simulink model "orion_casestudy_16"  (R2023a)
settings: Solver=VariableStepAuto  StartTime=0.0  StopTime=30  RelTol=1e-3
InitFcn:
  | RandStream.setGlobalStream(RandStream('mt19937ar','seed',sum(100*clock)));
undefined symbols (not defined in the file or in its folder): m, n
(part 2 of 4)

== stateflow chart orion_casestudy_16/Slave3 ==
  settings: updateMethod=CONTINUOUS
  state Connected
    entry:
    connStatus=2;
    state KeepAliveSendTimeout [parallel]
      settings: executionOrder=1
      state KeepAliveSend
      (default) -> KeepAliveSend
      KeepAliveSend -> KeepAliveSend [order 1] : after(delay_array(i)*5,msec)
          |  {OrionKeepAliveOut.data=0;
          | send(OrionKeepAliveOut);i = i + 1;}
      KeepAliveSend -> KeepAliveSend [order 2] : SendDataIn
          | {OrionAppDataOut.data=0;
          | send(OrionAppDataOut);}
    state KeepAliveRecieveTimeout [parallel]
      settings: executionOrder=2
      state KeepAlineRec
      (default) -> KeepAlineRec
      KeepAlineRec -> KeepAlineRec [order 2] : OrionKeepAliveIn
      KeepAlineRec -> KeepAlineRec [order 3] : OrionAppDataIn
  state Closed
    entry:
    connStatus=0;
  state Connecting
    entry:
    connStatus=1;
  Connected -> (junction 6) [order 2] : OrionConnRespIn
  Connected -> (junction 6) [order 3] : OrionConnReqIn
  (default) -> Closed : {i=1;}
  (junction 6) -> Closed
  Connected -> (junction 6) [order 1] : OrionConnConfIn
  KeepAlineRec -> Closed [order 1] : after(delay_array(i)*5,msec)
      | {i = i + 1;}
  Connecting -> (junction 36) [order 6] : OrionAppDataIn
  Connecting -> (junction 36) [order 5] : OrionConnReqIn
  (junction 36) -> Closed
  Connecting -> (junction 36) [order 4] : OrionConnRespIn
  Connecting -> (junction 36) [order 3] : OrionKeepAliveIn
  Closed -> Connecting : OrionConnReqIn
      | {OrionConnRespOut.data=0;
      | send(OrionConnRespOut);}
  Connecting -> Closed [order 1] : after(delay_array(i)*5,msec)
      | {i = i + 1;}
  Connecting -> Connected [order 2] : OrionConnConfIn{OrionConnConfOut.data=0;send(OrionConnConfOut);}
  data: OrionKeepAliveIn input; OrionConnConfOut output; OrionConnRespOut output; OrionKeepAliveOut output; OrionAppDataOut output; OrionAppDataIn input; OrionConnRespIn input; OrionConnReqIn input; OrionConnReqOut output size=1; connStatus output; SendDataIn local; OrionConnConfIn input; delay_array input; i local

== stateflow chart orion_casestudy_16/DelaySwitch41 ==
  state Operation
  state Sending
  (default) -> Operation : {i=0;}
  (junction 7) -> Operation [order 2]
  Sending -> Operation : after(delay_array(i),msec)
      | {receive(inMsg);outMsg.data=0;send(outMsg);}
  Operation -> (junction 7) : inMsg{i = i + 1;}
  (junction 7) -> Sending [order 1] : [switch_array(i)==0]
  data: switch_array input; delay_array input; outMsg output; inMsg input; i local

== stateflow chart orion_casestudy_16/DelaySwitch42 ==
  state Operation
  state Sending
  (default) -> Operation : {i=0;}
  (junction 7) -> Operation [order 2]
  Sending -> Operation : after(delay_array(i),msec)
      | {receive(inMsg);outMsg.data=0;send(outMsg);}
  Operation -> (junction 7) : inMsg{i = i + 1;}
  (junction 7) -> Sending [order 1] : [switch_array(i)==0]
  data: switch_array input; delay_array input; outMsg output; inMsg input; i local

== stateflow chart orion_casestudy_16/DelaySwitch43 ==
  state Operation
  state Sending
  (default) -> Operation : {i=0;}
  (junction 7) -> Operation [order 2]
  Sending -> Operation : after(delay_array(i),msec)
      | {receive(inMsg);outMsg.data=0;send(outMsg);}
  Operation -> (junction 7) : inMsg{i = i + 1;}
  (junction 7) -> Sending [order 1] : [switch_array(i)==0]
  data: switch_array input; delay_array input; outMsg output; inMsg input; i local

== stateflow chart orion_casestudy_16/DelaySwitch44 ==
  state Operation
  state Sending
  (default) -> Operation : {i=0;}
  (junction 7) -> Operation [order 2]
  Sending -> Operation : after(delay_array(i),msec)
      | {receive(inMsg);outMsg.data=0;send(outMsg);}
  Operation -> (junction 7) : inMsg{i = i + 1;}
  (junction 7) -> Sending [order 1] : [switch_array(i)==0]
  data: switch_array input; delay_array input; outMsg output; inMsg input; i local

== stateflow chart orion_casestudy_16/DelaySwitch45 ==
  state Operation
  state Sending
  (default) -> Operation : {i=0;}
  (junction 7) -> Operation [order 2]
  Sending -> Operation : after(delay_array(i),msec)
      | {receive(inMsg);outMsg.data=0;send(outMsg);}
  Operation -> (junction 7) : inMsg{i = i + 1;}
  (junction 7) -> Sending [order 1] : [switch_array(i)==0]
  data: switch_array input; delay_array input; outMsg output; inMsg input; i local

== stateflow chart orion_casestudy_16/DelaySwitch46 ==
  state Operation
  state Sending
  (default) -> Operation : {i=0;}
  (junction 7) -> Operation [order 2]
  Sending -> Operation : after(delay_array(i),msec)
      | {receive(inMsg);outMsg.data=0;send(outMsg);}
  Operation -> (junction 7) : inMsg{i = i + 1;}
  (junction 7) -> Sending [order 1] : [switch_array(i)==0]
  data: switch_array input; delay_array input; outMsg output; inMsg input; i local

== stateflow chart orion_casestudy_16/DelaySwitch47 ==
  state Operation
  state Sending
  (default) -> Operation : {i=0;}
  (junction 7) -> Operation [order 2]
  Sending -> Operation : after(delay_array(i),msec)
      | {receive(inMsg);outMsg.data=0;send(outMsg);}
  Operation -> (junction 7) : inMsg{i = i + 1;}
  (junction 7) -> Sending [order 1] : [switch_array(i)==0]
  data: switch_array input; delay_array input; outMsg output; inMsg input; i local

== stateflow chart orion_casestudy_16/DelaySwitch48 ==
  state Operation
  state Sending
  (default) -> Operation : {i=0;}
  (junction 7) -> Operation [order 2]
  Sending -> Operation : after(delay_array(i),msec)
      | {receive(inMsg);outMsg.data=0;send(outMsg);}
  Operation -> (junction 7) : inMsg{i = i + 1;}
  (junction 7) -> Sending [order 1] : [switch_array(i)==0]
  data: switch_array input; delay_array input; outMsg output; inMsg input; i local

== stateflow chart orion_casestudy_16/DelaySwitch49 ==
  state Operation
  state Sending
  (default) -> Operation : {i=0;}
  (junction 7) -> Operation [order 2]
  Sending -> Operation : after(delay_array(i),msec)
      | {receive(inMsg);outMsg.data=0;send(outMsg);}
  Operation -> (junction 7) : inMsg{i = i + 1;}
  (junction 7) -> Sending [order 1] : [switch_array(i)==0]
  data: switch_array input; delay_array input; outMsg output; inMsg input; i local

== stateflow chart orion_casestudy_16/DelaySwitch50 ==
  state Operation
  state Sending
  (default) -> Operation : {i=0;}
  (junction 7) -> Operation [order 2]
  Sending -> Operation : after(delay_array(i),msec)
      | {receive(inMsg);outMsg.data=0;send(outMsg);}
  Operation -> (junction 7) : inMsg{i = i + 1;}
  (junction 7) -> Sending [order 1] : [switch_array(i)==0]
  data: switch_array input; delay_array input; outMsg output; inMsg input; i local

== stateflow chart orion_casestudy_16/DelaySwitch51 ==
  state Operation
  state Sending
  (default) -> Operation : {i=0;}
  (junction 7) -> Operation [order 2]
  Sending -> Operation : after(delay_array(i),msec)
      | {receive(inMsg);outMsg.data=0;send(outMsg);}
  Operation -> (junction 7) : inMsg{i = i + 1;}
  (junction 7) -> Sending [order 1] : [switch_array(i)==0]
  data: switch_array input; delay_array input; outMsg output; inMsg input; i local

== stateflow chart orion_casestudy_16/DelaySwitch52 ==
  state Operation
  state Sending
  (default) -> Operation : {i=0;}
  (junction 7) -> Operation [order 2]
  Sending -> Operation : after(delay_array(i),msec)
      | {receive(inMsg);outMsg.data=0;send(outMsg);}
  Operation -> (junction 7) : inMsg{i = i + 1;}
  (junction 7) -> Sending [order 1] : [switch_array(i)==0]
  data: switch_array input; delay_array input; outMsg output; inMsg input; i local

== stateflow chart orion_casestudy_16/DelaySwitch53 ==
  state Operation
  state Sending
  (default) -> Operation : {i=0;}
  (junction 7) -> Operation [order 2]
  Sending -> Operation : after(delay_array(i),msec)
      | {receive(inMsg);outMsg.data=0;send(outMsg);}
  Operation -> (junction 7) : inMsg{i = i + 1;}
  (junction 7) -> Sending [order 1] : [switch_array(i)==0]
  data: switch_array input; delay_array input; outMsg output; inMsg input; i local

== stateflow chart orion_casestudy_16/DelaySwitch54 ==
  state Operation
  state Sending
  (default) -> Operation : {i=0;}
  (junction 7) -> Operation [order 2]
  Sending -> Operation : after(delay_array(i),msec)
      | {receive(inMsg);outMsg.data=0;send(outMsg);}
  Operation -> (junction 7) : inMsg{i = i + 1;}
  (junction 7) -> Sending [order 1] : [switch_array(i)==0]
  data: switch_array input; delay_array input; outMsg output; inMsg input; i local

== stateflow chart orion_casestudy_16/DelaySwitch55 ==
  state Operation
  state Sending
  (default) -> Operation : {i=0;}
  (junction 7) -> Operation [order 2]
  Sending -> Operation : after(delay_array(i),msec)
      | {receive(inMsg);outMsg.data=0;send(outMsg);}
  Operation -> (junction 7) : inMsg{i = i + 1;}
  (junction 7) -> Sending [order 1] : [switch_array(i)==0]
  data: switch_array input; delay_array input; outMsg output; inMsg input; i local

== stateflow chart orion_casestudy_16/DelaySwitch56 ==
  state Operation
  state Sending
  (default) -> Operation : {i=0;}
  (junction 7) -> Operation [order 2]
  Sending -> Operation : after(delay_array(i),msec)
      | {receive(inMsg);outMsg.data=0;send(outMsg);}
  Operation -> (junction 7) : inMsg{i = i + 1;}
  (junction 7) -> Sending [order 1] : [switch_array(i)==0]
  data: switch_array input; delay_array input; outMsg output; inMsg input; i local

== stateflow chart orion_casestudy_16/DelaySwitch57 ==
  state Operation
  state Sending
  (default) -> Operation : {i=0;}
  (junction 7) -> Operation [order 2]
  Sending -> Operation : after(delay_array(i),msec)
      | {receive(inMsg);outMsg.data=0;send(outMsg);}
  Operation -> (junction 7) : inMsg{i = i + 1;}
  (junction 7) -> Sending [order 1] : [switch_array(i)==0]
  data: switch_array input; delay_array input; outMsg output; inMsg input; i local

== stateflow chart orion_casestudy_16/DelaySwitch58 ==
  state Operation
  state Sending
  (default) -> Operation : {i=0;}
  (junction 7) -> Operation [order 2]
  Sending -> Operation : after(delay_array(i),msec)
      | {receive(inMsg);outMsg.data=0;send(outMsg);}
  Operation -> (junction 7) : inMsg{i = i + 1;}
  (junction 7) -> Sending [order 1] : [switch_array(i)==0]
  data: switch_array input; delay_array input; outMsg output; inMsg input; i local

== stateflow chart orion_casestudy_16/DelaySwitch59 ==
  state Operation
  state Sending
  (default) -> Operation : {i=0;}
  (junction 7) -> Operation [order 2]
  Sending -> Operation : after(delay_array(i),msec)
      | {receive(inMsg);outMsg.data=0;send(outMsg);}
  Operation -> (junction 7) : inMsg{i = i + 1;}
  (junction 7) -> Sending [order 1] : [switch_array(i)==0]
  data: switch_array input; delay_array input; outMsg output; inMsg input; i local

== stateflow chart orion_casestudy_16/DelaySwitch60 ==
  state Operation
  state Sending
  (default) -> Operation : {i=0;}
  (junction 7) -> Operation [order 2]
  Sending -> Operation : after(delay_array(i),msec)
      | {receive(inMsg);outMsg.data=0;send(outMsg);}
  Operation -> (junction 7) : inMsg{i = i + 1;}
  (junction 7) -> Sending [order 1] : [switch_array(i)==0]
  data: switch_array input; delay_array input; outMsg output; inMsg input; i local

== stateflow chart orion_casestudy_16/DelaySwitch61 ==
  state Operation
  state Sending
  (default) -> Operation : {i=0;}
  (junction 7) -> Operation [order 2]
  Sending -> Operation : after(delay_array(i),msec)
      | {receive(inMsg);outMsg.data=0;send(outMsg);}
  Operation -> (junction 7) : inMsg{i = i + 1;}
  (junction 7) -> Sending [order 1] : [switch_array(i)==0]
  data: switch_array input; delay_array input; outMsg output; inMsg input; i local

== stateflow chart orion_casestudy_16/DelaySwitch62 ==
  state Operation
  state Sending
  (default) -> Operation : {i=0;}
  (junction 7) -> Operation [order 2]
  Sending -> Operation : after(delay_array(i),msec)
      | {receive(inMsg);outMsg.data=0;send(outMsg);}
  Operation -> (junction 7) : inMsg{i = i + 1;}
  (junction 7) -> Sending [order 1] : [switch_array(i)==0]
  data: switch_array input; delay_array input; outMsg output; inMsg input; i local

== stateflow chart orion_casestudy_16/DelaySwitch3 ==
  state Operation
  state Sending
  (default) -> Operation : {i=0;}
  (junction 7) -> Operation [order 2]
  Sending -> Operation : after(delay_array(i),msec)
      | {receive(inMsg);outMsg.data=0;send(outMsg);}
  Operation -> (junction 7) : inMsg{i = i + 1;}
  (junction 7) -> Sending [order 1] : [switch_array(i)==0]
  data: switch_array input; delay_array input; outMsg output; inMsg input; i local

== stateflow chart orion_casestudy_16/DelaySwitch63 ==
  state Operation
  state Sending
  (default) -> Operation : {i=0;}
  (junction 7) -> Operation [order 2]
  Sending -> Operation : after(delay_array(i),msec)
      | {receive(inMsg);outMsg.data=0;send(outMsg);}
  Operation -> (junction 7) : inMsg{i = i + 1;}
  (junction 7) -> Sending [order 1] : [switch_array(i)==0]
  data: switch_array input; delay_array input; outMsg output; inMsg input; i local

== stateflow chart orion_casestudy_16/DelaySwitch64 ==
  state Operation
  state Sending
  (default) -> Operation : {i=0;}
  (junction 7) -> Operation [order 2]
  Sending -> Operation : after(delay_array(i),msec)
      | {receive(inMsg);outMsg.data=0;send(outMsg);}
  Operation -> (junction 7) : inMsg{i = i + 1;}
  (junction 7) -> Sending [order 1] : [switch_array(i)==0]
  data: switch_array input; delay_array input; outMsg output; inMsg input; i local

== stateflow chart orion_casestudy_16/DelaySwitch65 ==
  state Operation
  state Sending
  (default) -> Operation : {i=0;}
  (junction 7) -> Operation [order 2]
  Sending -> Operation : after(delay_array(i),msec)
      | {receive(inMsg);outMsg.data=0;send(outMsg);}
  Operation -> (junction 7) : inMsg{i = i + 1;}
  (junction 7) -> Sending [order 1] : [switch_array(i)==0]
  data: switch_array input; delay_array input; outMsg output; inMsg input; i local

== stateflow chart orion_casestudy_16/DelaySwitch66 ==
  state Operation
  state Sending
  (default) -> Operation : {i=0;}
  (junction 7) -> Operation [order 2]
  Sending -> Operation : after(delay_array(i),msec)
      | {receive(inMsg);outMsg.data=0;send(outMsg);}
  Operation -> (junction 7) : inMsg{i = i + 1;}
  (junction 7) -> Sending [order 1] : [switch_array(i)==0]
  data: switch_array input; delay_array input; outMsg output; inMsg input; i local

== stateflow chart orion_casestudy_16/DelaySwitch67 ==
  state Operation
  state Sending
  (default) -> Operation : {i=0;}
  (junction 7) -> Operation [order 2]
  Sending -> Operation : after(delay_array(i),msec)
      | {receive(inMsg);outMsg.data=0;send(outMsg);}
  Operation -> (junction 7) : inMsg{i = i + 1;}
  (junction 7) -> Sending [order 1] : [switch_array(i)==0]
  data: switch_array input; delay_array input; outMsg output; inMsg input; i local

== stateflow chart orion_casestudy_16/DelaySwitch68 ==
  state Operation
  state Sending
  (default) -> Operation : {i=0;}
  (junction 7) -> Operation [order 2]
  Sending -> Operation : after(delay_array(i),msec)
      | {receive(inMsg);outMsg.data=0;send(outMsg);}
  Operation -> (junction 7) : inMsg{i = i + 1;}
  (junction 7) -> Sending [order 1] : [switch_array(i)==0]
  data: switch_array input; delay_array input; outMsg output; inMsg input; i local

== stateflow chart orion_casestudy_16/DelaySwitch69 ==
  state Operation
  state Sending
  (default) -> Operation : {i=0;}
  (junction 7) -> Operation [order 2]
  Sending -> Operation : after(delay_array(i),msec)
      | {receive(inMsg);outMsg.data=0;send(outMsg);}
  Operation -> (junction 7) : inMsg{i = i + 1;}
  (junction 7) -> Sending [order 1] : [switch_array(i)==0]
  data: switch_array input; delay_array input; outMsg output; inMsg input; i local

== stateflow chart orion_casestudy_16/DelaySwitch70 ==
  state Operation
  state Sending
  (default) -> Operation : {i=0;}
  (junction 7) -> Operation [order 2]
  Sending -> Operation : after(delay_array(i),msec)
      | {receive(inMsg);outMsg.data=0;send(outMsg);}
  Operation -> (junction 7) : inMsg{i = i + 1;}
  (junction 7) -> Sending [order 1] : [switch_array(i)==0]
  data: switch_array input; delay_array input; outMsg output; inMsg input; i local

== stateflow chart orion_casestudy_16/DelaySwitch71 ==
  state Operation
  state Sending
  (default) -> Operation : {i=0;}
  (junction 7) -> Operation [order 2]
  Sending -> Operation : after(delay_array(i),msec)
      | {receive(inMsg);outMsg.data=0;send(outMsg);}
  Operation -> (junction 7) : inMsg{i = i + 1;}
  (junction 7) -> Sending [order 1] : [switch_array(i)==0]
  data: switch_array input; delay_array input; outMsg output; inMsg input; i local

== stateflow chart orion_casestudy_16/DelaySwitch72 ==
  state Operation
  state Sending
  (default) -> Operation : {i=0;}
  (junction 7) -> Operation [order 2]
  Sending -> Operation : after(delay_array(i),msec)
      | {receive(inMsg);outMsg.data=0;send(outMsg);}
  Operation -> (junction 7) : inMsg{i = i + 1;}
  (junction 7) -> Sending [order 1] : [switch_array(i)==0]
  data: switch_array input; delay_array input; outMsg output; inMsg input; i local

== stateflow chart orion_casestudy_16/DelaySwitch4 ==
  state Operation
  state Sending
  (default) -> Operation : {i=0;}
  (junction 7) -> Operation [order 2]
  Sending -> Operation : after(delay_array(i),msec)
      | {receive(inMsg);outMsg.data=0;send(outMsg);}
  Operation -> (junction 7) : inMsg{i = i + 1;}
  (junction 7) -> Sending [order 1] : [switch_array(i)==0]
  data: switch_array input; delay_array input; outMsg output; inMsg input; i local

== stateflow chart orion_casestudy_16/DelaySwitch73 ==
  state Operation
  state Sending
  (default) -> Operation : {i=0;}
  (junction 7) -> Operation [order 2]
  Sending -> Operation : after(delay_array(i),msec)
      | {receive(inMsg);outMsg.data=0;send(outMsg);}
  Operation -> (junction 7) : inMsg{i = i + 1;}
  (junction 7) -> Sending [order 1] : [switch_array(i)==0]
  data: switch_array input; delay_array input; outMsg output; inMsg input; i local

== stateflow chart orion_casestudy_16/DelaySwitch74 ==
  state Operation
  state Sending
  (default) -> Operation : {i=0;}
  (junction 7) -> Operation [order 2]
  Sending -> Operation : after(delay_array(i),msec)
      | {receive(inMsg);outMsg.data=0;send(outMsg);}
  Operation -> (junction 7) : inMsg{i = i + 1;}
  (junction 7) -> Sending [order 1] : [switch_array(i)==0]
  data: switch_array input; delay_array input; outMsg output; inMsg input; i local

== stateflow chart orion_casestudy_16/DelaySwitch75 ==
  state Operation
  state Sending
  (default) -> Operation : {i=0;}
  (junction 7) -> Operation [order 2]
  Sending -> Operation : after(delay_array(i),msec)
      | {receive(inMsg);outMsg.data=0;send(outMsg);}
  Operation -> (junction 7) : inMsg{i = i + 1;}
  (junction 7) -> Sending [order 1] : [switch_array(i)==0]
  data: switch_array input; delay_array input; outMsg output; inMsg input; i local

== stateflow chart orion_casestudy_16/DelaySwitch76 ==
  state Operation
  state Sending
  (default) -> Operation : {i=0;}
  (junction 7) -> Operation [order 2]
  Sending -> Operation : after(delay_array(i),msec)
      | {receive(inMsg);outMsg.data=0;send(outMsg);}
  Operation -> (junction 7) : inMsg{i = i + 1;}
  (junction 7) -> Sending [order 1] : [switch_array(i)==0]
  data: switch_array input; delay_array input; outMsg output; inMsg input; i local

== stateflow chart orion_casestudy_16/DelaySwitch77 ==
  state Operation
  state Sending
  (default) -> Operation : {i=0;}
  (junction 7) -> Operation [order 2]
  Sending -> Operation : after(delay_array(i),msec)
      | {receive(inMsg);outMsg.data=0;send(outMsg);}
  Operation -> (junction 7) : inMsg{i = i + 1;}
  (junction 7) -> Sending [order 1] : [switch_array(i)==0]
  data: switch_array input; delay_array input; outMsg output; inMsg input; i local

== stateflow chart orion_casestudy_16/DelaySwitch78 ==
  state Operation
  state Sending
  (default) -> Operation : {i=0;}
  (junction 7) -> Operation [order 2]
  Sending -> Operation : after(delay_array(i),msec)
      | {receive(inMsg);outMsg.data=0;send(outMsg);}
  Operation -> (junction 7) : inMsg{i = i + 1;}
  (junction 7) -> Sending [order 1] : [switch_array(i)==0]
  data: switch_array input; delay_array input; outMsg output; inMsg input; i local

== stateflow chart orion_casestudy_16/DelaySwitch79 ==
  state Operation
  state Sending
  (default) -> Operation : {i=0;}
  (junction 7) -> Operation [order 2]
  Sending -> Operation : after(delay_array(i),msec)
      | {receive(inMsg);outMsg.data=0;send(outMsg);}
  Operation -> (junction 7) : inMsg{i = i + 1;}
  (junction 7) -> Sending [order 1] : [switch_array(i)==0]
  data: switch_array input; delay_array input; outMsg output; inMsg input; i local

== stateflow chart orion_casestudy_16/DelaySwitch80 ==
  state Operation
  state Sending
  (default) -> Operation : {i=0;}
  (junction 7) -> Operation [order 2]
  Sending -> Operation : after(delay_array(i),msec)
      | {receive(inMsg);outMsg.data=0;send(outMsg);}
  Operation -> (junction 7) : inMsg{i = i + 1;}
  (junction 7) -> Sending [order 1] : [switch_array(i)==0]
  data: switch_array input; delay_array input; outMsg output; inMsg input; i local

== stateflow chart orion_casestudy_16/Master4 ==
  settings: updateMethod=CONTINUOUS
  state Connected
    entry:
    connStatus=2;
    state KeepAliveSendTimeout [parallel]
      settings: executionOrder=1
      state KeepAliveSend
      (default) -> KeepAliveSend
      KeepAliveSend -> KeepAliveSend [order 1] : after(delay_array(i)*5,msec)
          | {OrionKeepAliveOut.data=0;
          | send(OrionKeepAliveOut);
          | i = i + 1;}
      KeepAliveSend -> KeepAliveSend [order 2] : SendDataIn
          | {OrionAppDataOut.data=0;
          | send(OrionAppDataOut);}
    state KeepAliveRecieveTimeout [parallel]
      settings: executionOrder=2
      state KeepAlineRec
      (default) -> KeepAlineRec
      KeepAlineRec -> KeepAlineRec [order 2] : OrionKeepAliveIn
      KeepAlineRec -> KeepAlineRec [order 3] : OrionAppDataIn
  state Closed
    entry:
    connStatus=0;
  state Connecting
    entry:
    connStatus=1;
  Connected -> (junction 6) [order 1] : OrionConnConfIn
  (default) -> Closed : {i=1;}
  Connected -> (junction 6) [order 2] : OrionConnRespIn
  Connected -> (junction 6) [order 3] : OrionConnReqIn
  (junction 6) -> Closed
  KeepAlineRec -> Closed [order 1] : after(delay_array(i)*5,msec)
      | {i = i + 1;}
  Connecting -> (junction 36) [order 5] : OrionConnReqIn
  (junction 36) -> Closed
  Connecting -> (junction 36) [order 4] : OrionConnRespIn
  Connecting -> (junction 36) [order 2] : OrionKeepAliveIn
  Connecting -> Closed [order 3] : after(delay_array(i)*5,msec)
      | {i = i + 1;}
  Closed -> Connecting [order 2] : after(delay_array(i)*5,msec)
      | {OrionConnReqOut.data=0;send(OrionConnReqOut);i = i + 1;}
  Closed -> Connecting [order 1] : OrionConnReqIn
      | {OrionConnRespOut.data=0;send(OrionConnRespOut);}
  Connecting -> Connected [order 1] : OrionConnRespIn
      | {OrionConnConfOut.data=0;
      | send(OrionConnConfOut);}
  data: delay_array input; OrionKeepAliveOut output; OrionKeepAliveIn input; OrionConnConfOut output; OrionConnConfIn input; OrionConnRespOut output; OrionAppDataOut output; OrionAppDataIn input; OrionConnRespIn input; OrionConnReqIn input; OrionConnReqOut output; connStatus output; SendDataIn local; i local

== stateflow chart orion_casestudy_16/DelaySwitch5 ==
  state Operation
  state Sending
  (default) -> Operation : {i=0;}
  (junction 7) -> Operation [order 2]
  Sending -> Operation : after(delay_array(i),msec)
      | {receive(inMsg);outMsg.data=0;send(outMsg);}
  Operation -> (junction 7) : inMsg{i = i + 1;}
  (junction 7) -> Sending [order 1] : [switch_array(i)==0]
  data: switch_array input; delay_array input; outMsg output; inMsg input; i local

== stateflow chart orion_casestudy_16/Master5 ==
  settings: updateMethod=CONTINUOUS
  state Connected
    entry:
    connStatus=2;
    state KeepAliveSendTimeout [parallel]
      settings: executionOrder=1
      state KeepAliveSend
      (default) -> KeepAliveSend
      KeepAliveSend -> KeepAliveSend [order 1] : after(delay_array(i)*5,msec)
          | {OrionKeepAliveOut.data=0;
          | send(OrionKeepAliveOut);
          | i = i + 1;}
      KeepAliveSend -> KeepAliveSend [order 2] : SendDataIn
          | {OrionAppDataOut.data=0;
          | send(OrionAppDataOut);}
    state KeepAliveRecieveTimeout [parallel]
      settings: executionOrder=2
      state KeepAlineRec
      (default) -> KeepAlineRec
      KeepAlineRec -> KeepAlineRec [order 2] : OrionKeepAliveIn
      KeepAlineRec -> KeepAlineRec [order 3] : OrionAppDataIn
  state Closed
    entry:
    connStatus=0;
  state Connecting
    entry:
    connStatus=1;
  Connected -> (junction 6) [order 1] : OrionConnConfIn
  (default) -> Closed : {i=1;}
  Connected -> (junction 6) [order 2] : OrionConnRespIn
  Connected -> (junction 6) [order 3] : OrionConnReqIn
  (junction 6) -> Closed
  KeepAlineRec -> Closed [order 1] : after(delay_array(i)*5,msec)
      | {i = i + 1;}
  Connecting -> (junction 36) [order 5] : OrionConnReqIn
  (junction 36) -> Closed
  Connecting -> (junction 36) [order 4] : OrionConnRespIn
  Connecting -> (junction 36) [order 2] : OrionKeepAliveIn
  Connecting -> Closed [order 3] : after(delay_array(i)*5,msec)
      | {i = i + 1;}
  Closed -> Connecting [order 2] : after(delay_array(i)*5,msec)
      | {OrionConnReqOut.data=0;send(OrionConnReqOut);i = i + 1;}
  Closed -> Connecting [order 1] : OrionConnReqIn
      | {OrionConnRespOut.data=0;send(OrionConnRespOut);}
  Connecting -> Connected [order 1] : OrionConnRespIn
      | {OrionConnConfOut.data=0;
      | send(OrionConnConfOut);}
  data: delay_array input; OrionKeepAliveOut output; OrionKeepAliveIn input; OrionConnConfOut output; OrionConnConfIn input; OrionConnRespOut output; OrionAppDataOut output; OrionAppDataIn input; OrionConnRespIn input; OrionConnReqIn input; OrionConnReqOut output; connStatus output; SendDataIn local; i local

== stateflow chart orion_casestudy_16/Master6 ==
  settings: updateMethod=CONTINUOUS
  state Connected
    entry:
    connStatus=2;
    state KeepAliveSendTimeout [parallel]
      settings: executionOrder=1
      state KeepAliveSend
      (default) -> KeepAliveSend
      KeepAliveSend -> KeepAliveSend [order 1] : after(delay_array(i)*5,msec)
          | {OrionKeepAliveOut.data=0;
          | send(OrionKeepAliveOut);
          | i = i + 1;}
      KeepAliveSend -> KeepAliveSend [order 2] : SendDataIn
          | {OrionAppDataOut.data=0;
          | send(OrionAppDataOut);}
    state KeepAliveRecieveTimeout [parallel]
      settings: executionOrder=2
      state KeepAlineRec
      (default) -> KeepAlineRec
      KeepAlineRec -> KeepAlineRec [order 2] : OrionKeepAliveIn
      KeepAlineRec -> KeepAlineRec [order 3] : OrionAppDataIn
  state Closed
    entry:
    connStatus=0;
  state Connecting
    entry:
    connStatus=1;
  Connected -> (junction 6) [order 1] : OrionConnConfIn
  (default) -> Closed : {i=1;}
  Connected -> (junction 6) [order 2] : OrionConnRespIn
  Connected -> (junction 6) [order 3] : OrionConnReqIn
  (junction 6) -> Closed
  KeepAlineRec -> Closed [order 1] : after(delay_array(i)*5,msec)
      | {i = i + 1;}
  Connecting -> (junction 36) [order 5] : OrionConnReqIn
  (junction 36) -> Closed
  Connecting -> (junction 36) [order 4] : OrionConnRespIn
  Connecting -> (junction 36) [order 2] : OrionKeepAliveIn
  Connecting -> Closed [order 3] : after(delay_array(i)*5,msec)
      | {i = i + 1;}
  Closed -> Connecting [order 2] : after(delay_array(i)*5,msec)
      | {OrionConnReqOut.data=0;send(OrionConnReqOut);i = i + 1;}
  Closed -> Connecting [order 1] : OrionConnReqIn
      | {OrionConnRespOut.data=0;send(OrionConnRespOut);}
  Connecting -> Connected [order 1] : OrionConnRespIn
      | {OrionConnConfOut.data=0;
      | send(OrionConnConfOut);}
  data: delay_array input; OrionKeepAliveOut output; OrionKeepAliveIn input; OrionConnConfOut output; OrionConnConfIn input; OrionConnRespOut output; OrionAppDataOut output; OrionAppDataIn input; OrionConnRespIn input; OrionConnReqIn input; OrionConnReqOut output; connStatus output; SendDataIn local; i local

== stateflow chart orion_casestudy_16/Master7 ==
  settings: updateMethod=CONTINUOUS
  state Connected
    entry:
    connStatus=2;
    state KeepAliveSendTimeout [parallel]
      settings: executionOrder=1
      state KeepAliveSend
      (default) -> KeepAliveSend
      KeepAliveSend -> KeepAliveSend [order 1] : after(delay_array(i)*5,msec)
          | {OrionKeepAliveOut.data=0;
          | send(OrionKeepAliveOut);
          | i = i + 1;}
      KeepAliveSend -> KeepAliveSend [order 2] : SendDataIn
          | {OrionAppDataOut.data=0;
          | send(OrionAppDataOut);}
    state KeepAliveRecieveTimeout [parallel]
      settings: executionOrder=2
      state KeepAlineRec
      (default) -> KeepAlineRec
      KeepAlineRec -> KeepAlineRec [order 2] : OrionKeepAliveIn
      KeepAlineRec -> KeepAlineRec [order 3] : OrionAppDataIn
  state Closed
    entry:
    connStatus=0;
  state Connecting
    entry:
    connStatus=1;
  Connected -> (junction 6) [order 1] : OrionConnConfIn
  (default) -> Closed : {i=1;}
  Connected -> (junction 6) [order 2] : OrionConnRespIn
  Connected -> (junction 6) [order 3] : OrionConnReqIn
  (junction 6) -> Closed
  KeepAlineRec -> Closed [order 1] : after(delay_array(i)*5,msec)
      | {i = i + 1;}
  Connecting -> (junction 36) [order 5] : OrionConnReqIn
  (junction 36) -> Closed
  Connecting -> (junction 36) [order 4] : OrionConnRespIn
  Connecting -> (junction 36) [order 2] : OrionKeepAliveIn
  Connecting -> Closed [order 3] : after(delay_array(i)*5,msec)
      | {i = i + 1;}
  Closed -> Connecting [order 2] : after(delay_array(i)*5,msec)
      | {OrionConnReqOut.data=0;send(OrionConnReqOut);i = i + 1;}
  Closed -> Connecting [order 1] : OrionConnReqIn
      | {OrionConnRespOut.data=0;send(OrionConnRespOut);}
  Connecting -> Connected [order 1] : OrionConnRespIn
      | {OrionConnConfOut.data=0;
      | send(OrionConnConfOut);}
  data: delay_array input; OrionKeepAliveOut output; OrionKeepAliveIn input; OrionConnConfOut output; OrionConnConfIn input; OrionConnRespOut output; OrionAppDataOut output; OrionAppDataIn input; OrionConnRespIn input; OrionConnReqIn input; OrionConnReqOut output; connStatus output; SendDataIn local; i local

== stateflow chart orion_casestudy_16/DelaySwitch6 ==
  state Operation
  state Sending
  (default) -> Operation : {i=0;}
  (junction 7) -> Operation [order 2]
  Sending -> Operation : after(delay_array(i),msec)
      | {receive(inMsg);outMsg.data=0;send(outMsg);}
  Operation -> (junction 7) : inMsg{i = i + 1;}
  (junction 7) -> Sending [order 1] : [switch_array(i)==0]
  data: switch_array input; delay_array input; outMsg output; inMsg input; i local

== stateflow chart orion_casestudy_16/Slave4 ==
  settings: updateMethod=CONTINUOUS
  state Connected
    entry:
    connStatus=2;
    state KeepAliveSendTimeout [parallel]
      settings: executionOrder=1
      state KeepAliveSend
      (default) -> KeepAliveSend
      KeepAliveSend -> KeepAliveSend [order 1] : after(delay_array(i)*5,msec)
          |  {OrionKeepAliveOut.data=0;
          | send(OrionKeepAliveOut);i = i + 1;}
      KeepAliveSend -> KeepAliveSend [order 2] : SendDataIn
          | {OrionAppDataOut.data=0;
          | send(OrionAppDataOut);}
    state KeepAliveRecieveTimeout [parallel]
      settings: executionOrder=2
      state KeepAlineRec
      (default) -> KeepAlineRec
      KeepAlineRec -> KeepAlineRec [order 2] : OrionKeepAliveIn
      KeepAlineRec -> KeepAlineRec [order 3] : OrionAppDataIn
  state Closed
    entry:
    connStatus=0;
  state Connecting
    entry:
    connStatus=1;
  Connected -> (junction 6) [order 2] : OrionConnRespIn
  Connected -> (junction 6) [order 3] : OrionConnReqIn
  (default) -> Closed : {i=1;}
  (junction 6) -> Closed
  Connected -> (junction 6) [order 1] : OrionConnConfIn
  KeepAlineRec -> Closed [order 1] : after(delay_array(i)*5,msec)
      | {i = i + 1;}
  Connecting -> (junction 36) [order 6] : OrionAppDataIn
  Connecting -> (junction 36) [order 5] : OrionConnReqIn
  (junction 36) -> Closed
  Connecting -> (junction 36) [order 4] : OrionConnRespIn
  Connecting -> (junction 36) [order 3] : OrionKeepAliveIn
  Closed -> Connecting : OrionConnReqIn
      | {OrionConnRespOut.data=0;
      | send(OrionConnRespOut);}
  Connecting -> Closed [order 1] : after(delay_array(i)*5,msec)
      | {i = i + 1;}
  Connecting -> Connected [order 2] : OrionConnConfIn{OrionConnConfOut.data=0;send(OrionConnConfOut);}
  data: OrionKeepAliveIn input; OrionConnConfOut output; OrionConnRespOut output; OrionKeepAliveOut output; OrionAppDataOut output; OrionAppDataIn input; OrionConnRespIn input; OrionConnReqIn input; OrionConnReqOut output size=1; connStatus output; SendDataIn local; OrionConnConfIn input; delay_array input; i local

== stateflow chart orion_casestudy_16/Slave5 ==
  settings: updateMethod=CONTINUOUS
  state Connected
    entry:
    connStatus=2;
    state KeepAliveSendTimeout [parallel]
      settings: executionOrder=1
      state KeepAliveSend
      (default) -> KeepAliveSend
      KeepAliveSend -> KeepAliveSend [order 1] : after(delay_array(i)*5,msec)
          |  {OrionKeepAliveOut.data=0;
          | send(OrionKeepAliveOut);i = i + 1;}
      KeepAliveSend -> KeepAliveSend [order 2] : SendDataIn
          | {OrionAppDataOut.data=0;
          | send(OrionAppDataOut);}
    state KeepAliveRecieveTimeout [parallel]
      settings: executionOrder=2
      state KeepAlineRec
      (default) -> KeepAlineRec
      KeepAlineRec -> KeepAlineRec [order 2] : OrionKeepAliveIn
      KeepAlineRec -> KeepAlineRec [order 3] : OrionAppDataIn
  state Closed
    entry:
    connStatus=0;
  state Connecting
    entry:
    connStatus=1;
  Connected -> (junction 6) [order 2] : OrionConnRespIn
  Connected -> (junction 6) [order 3] : OrionConnReqIn
  (default) -> Closed : {i=1;}
  (junction 6) -> Closed
  Connected -> (junction 6) [order 1] : OrionConnConfIn
  KeepAlineRec -> Closed [order 1] : after(delay_array(i)*5,msec)
      | {i = i + 1;}
  Connecting -> (junction 36) [order 6] : OrionAppDataIn
  Connecting -> (junction 36) [order 5] : OrionConnReqIn
  (junction 36) -> Closed
  Connecting -> (junction 36) [order 4] : OrionConnRespIn
  Connecting -> (junction 36) [order 3] : OrionKeepAliveIn
  Closed -> Connecting : OrionConnReqIn
      | {OrionConnRespOut.data=0;
      | send(OrionConnRespOut);}
  Connecting -> Closed [order 1] : after(delay_array(i)*5,msec)
      | {i = i + 1;}
  Connecting -> Connected [order 2] : OrionConnConfIn{OrionConnConfOut.data=0;send(OrionConnConfOut);}
  data: OrionKeepAliveIn input; OrionConnConfOut output; OrionConnRespOut output; OrionKeepAliveOut output; OrionAppDataOut output; OrionAppDataIn input; OrionConnRespIn input; OrionConnReqIn input; OrionConnReqOut output size=1; connStatus output; SendDataIn local; OrionConnConfIn input; delay_array input; i local

== stateflow chart orion_casestudy_16/Slave6 ==
  settings: updateMethod=CONTINUOUS
  state Connected
    entry:
    connStatus=2;
    state KeepAliveSendTimeout [parallel]
      settings: executionOrder=1
      state KeepAliveSend
      (default) -> KeepAliveSend
      KeepAliveSend -> KeepAliveSend [order 1] : after(delay_array(i)*5,msec)
          |  {OrionKeepAliveOut.data=0;
          | send(OrionKeepAliveOut);i = i + 1;}
      KeepAliveSend -> KeepAliveSend [order 2] : SendDataIn
          | {OrionAppDataOut.data=0;
          | send(OrionAppDataOut);}
    state KeepAliveRecieveTimeout [parallel]
      settings: executionOrder=2
      state KeepAlineRec
      (default) -> KeepAlineRec
      KeepAlineRec -> KeepAlineRec [order 2] : OrionKeepAliveIn
      KeepAlineRec -> KeepAlineRec [order 3] : OrionAppDataIn
  state Closed
    entry:
    connStatus=0;
  state Connecting
    entry:
    connStatus=1;
  Connected -> (junction 6) [order 2] : OrionConnRespIn
  Connected -> (junction 6) [order 3] : OrionConnReqIn
  (default) -> Closed : {i=1;}
  (junction 6) -> Closed
  Connected -> (junction 6) [order 1] : OrionConnConfIn
  KeepAlineRec -> Closed [order 1] : after(delay_array(i)*5,msec)
      | {i = i + 1;}
  Connecting -> (junction 36) [order 6] : OrionAppDataIn
  Connecting -> (junction 36) [order 5] : OrionConnReqIn
  (junction 36) -> Closed
  Connecting -> (junction 36) [order 4] : OrionConnRespIn
  Connecting -> (junction 36) [order 3] : OrionKeepAliveIn
  Closed -> Connecting : OrionConnReqIn
      | {OrionConnRespOut.data=0;
      | send(OrionConnRespOut);}
  Connecting -> Closed [order 1] : after(delay_array(i)*5,msec)
      | {i = i + 1;}
  Connecting -> Connected [order 2] : OrionConnConfIn{OrionConnConfOut.data=0;send(OrionConnConfOut);}
  data: OrionKeepAliveIn input; OrionConnConfOut output; OrionConnRespOut output; OrionKeepAliveOut output; OrionAppDataOut output; OrionAppDataIn input; OrionConnRespIn input; OrionConnReqIn input; OrionConnReqOut output size=1; connStatus output; SendDataIn local; OrionConnConfIn input; delay_array input; i local

== stateflow chart orion_casestudy_16/Slave7 ==
  settings: updateMethod=CONTINUOUS
  state Connected
    entry:
    connStatus=2;
    state KeepAliveSendTimeout [parallel]
      settings: executionOrder=1
      state KeepAliveSend
      (default) -> KeepAliveSend
      KeepAliveSend -> KeepAliveSend [order 1] : after(delay_array(i)*5,msec)
          |  {OrionKeepAliveOut.data=0;
          | send(OrionKeepAliveOut);i = i + 1;}
      KeepAliveSend -> KeepAliveSend [order 2] : SendDataIn
          | {OrionAppDataOut.data=0;
          | send(OrionAppDataOut);}
    state KeepAliveRecieveTimeout [parallel]
      settings: executionOrder=2
      state KeepAlineRec
      (default) -> KeepAlineRec
      KeepAlineRec -> KeepAlineRec [order 2] : OrionKeepAliveIn
      KeepAlineRec -> KeepAlineRec [order 3] : OrionAppDataIn
  state Closed
    entry:
    connStatus=0;
  state Connecting
    entry:
    connStatus=1;
  Connected -> (junction 6) [order 2] : OrionConnRespIn
  Connected -> (junction 6) [order 3] : OrionConnReqIn
  (default) -> Closed : {i=1;}
  (junction 6) -> Closed
  Connected -> (junction 6) [order 1] : OrionConnConfIn
  KeepAlineRec -> Closed [order 1] : after(delay_array(i)*5,msec)
      | {i = i + 1;}
  Connecting -> (junction 36) [order 6] : OrionAppDataIn
  Connecting -> (junction 36) [order 5] : OrionConnReqIn
  (junction 36) -> Closed
  Connecting -> (junction 36) [order 4] : OrionConnRespIn
  Connecting -> (junction 36) [order 3] : OrionKeepAliveIn
  Closed -> Connecting : OrionConnReqIn
      | {OrionConnRespOut.data=0;
      | send(OrionConnRespOut);}
  Connecting -> Closed [order 1] : after(delay_array(i)*5,msec)
      | {i = i + 1;}
  Connecting -> Connected [order 2] : OrionConnConfIn{OrionConnConfOut.data=0;send(OrionConnConfOut);}
  data: OrionKeepAliveIn input; OrionConnConfOut output; OrionConnRespOut output; OrionKeepAliveOut output; OrionAppDataOut output; OrionAppDataIn input; OrionConnRespIn input; OrionConnReqIn input; OrionConnReqOut output size=1; connStatus output; SendDataIn local; OrionConnConfIn input; delay_array input; i local

== stateflow chart orion_casestudy_16/Slave ==
  settings: updateMethod=CONTINUOUS
  state Connected
    entry:
    connStatus=2;
    state KeepAliveSendTimeout [parallel]
      settings: executionOrder=1
      state KeepAliveSend
      (default) -> KeepAliveSend
      KeepAliveSend -> KeepAliveSend [order 1] : after(delay_array(i)*5,msec)
          |  {OrionKeepAliveOut.data=0;
          | send(OrionKeepAliveOut);i = i + 1;}
      KeepAliveSend -> KeepAliveSend [order 2] : SendDataIn
          | {OrionAppDataOut.data=0;
          | send(OrionAppDataOut);}
    state KeepAliveRecieveTimeout [parallel]
      settings: executionOrder=2
      state KeepAlineRec
      (default) -> KeepAlineRec
      KeepAlineRec -> KeepAlineRec [order 2] : OrionKeepAliveIn
      KeepAlineRec -> KeepAlineRec [order 3] : OrionAppDataIn
  state Closed
    entry:
    connStatus=0;
  state Connecting
    entry:
    connStatus=1;
  Connected -> (junction 6) [order 2] : OrionConnRespIn
  Connected -> (junction 6) [order 3] : OrionConnReqIn
  (default) -> Closed : {i=1;}
  (junction 6) -> Closed
  Connected -> (junction 6) [order 1] : OrionConnConfIn
  KeepAlineRec -> Closed [order 1] : after(delay_array(i)*5,msec)
      | {i = i + 1;}
  Connecting -> (junction 36) [order 6] : OrionAppDataIn
  Connecting -> (junction 36) [order 5] : OrionConnReqIn
  (junction 36) -> Closed
  Connecting -> (junction 36) [order 4] : OrionConnRespIn
  Connecting -> (junction 36) [order 3] : OrionKeepAliveIn
  Closed -> Connecting : OrionConnReqIn
      | {OrionConnRespOut.data=0;
      | send(OrionConnRespOut);}
  Connecting -> Closed [order 1] : after(delay_array(i)*5,msec)
      | {i = i + 1;}
  Connecting -> Connected [order 2] : OrionConnConfIn{OrionConnConfOut.data=0;send(OrionConnConfOut);}
  data: OrionKeepAliveIn input; OrionConnConfOut output; OrionConnRespOut output; OrionKeepAliveOut output; OrionAppDataOut output; OrionAppDataIn input; OrionConnRespIn input; OrionConnReqIn input; OrionConnReqOut output size=1; connStatus output; SendDataIn local; OrionConnConfIn input; delay_array input; i local

== stateflow chart orion_casestudy_16/DelaySwitch100 ==
  state Operation
  state Sending
  (default) -> Operation : {i=0;}
  (junction 7) -> Operation [order 2]
  Sending -> Operation : after(delay_array(i),msec)
      | {receive(inMsg);outMsg.data=0;send(outMsg);}
  Operation -> (junction 7) : inMsg{i = i + 1;}
  (junction 7) -> Sending [order 1] : [switch_array(i)==0]
  data: switch_array input; delay_array input; outMsg output; inMsg input; i local

== stateflow chart orion_casestudy_16/DelaySwitch101 ==
  state Operation
  state Sending
  (default) -> Operation : {i=0;}
  (junction 7) -> Operation [order 2]
  Sending -> Operation : after(delay_array(i),msec)
      | {receive(inMsg);outMsg.data=0;send(outMsg);}
  Operation -> (junction 7) : inMsg{i = i + 1;}
  (junction 7) -> Sending [order 1] : [switch_array(i)==0]
  data: switch_array input; delay_array input; outMsg output; inMsg input; i local

== stateflow chart orion_casestudy_16/DelaySwitch102 ==
  state Operation
  state Sending
  (default) -> Operation : {i=0;}
  (junction 7) -> Operation [order 2]
  Sending -> Operation : after(delay_array(i),msec)
      | {receive(inMsg);outMsg.data=0;send(outMsg);}
  Operation -> (junction 7) : inMsg{i = i + 1;}
  (junction 7) -> Sending [order 1] : [switch_array(i)==0]
  data: switch_array input; delay_array input; outMsg output; inMsg input; i local

== stateflow chart orion_casestudy_16/DelaySwitch103 ==
  state Operation
  state Sending
  (default) -> Operation : {i=0;}
  (junction 7) -> Operation [order 2]
  Sending -> Operation : after(delay_array(i),msec)
      | {receive(inMsg);outMsg.data=0;send(outMsg);}
  Operation -> (junction 7) : inMsg{i = i + 1;}
  (junction 7) -> Sending [order 1] : [switch_array(i)==0]
  data: switch_array input; delay_array input; outMsg output; inMsg input; i local

== stateflow chart orion_casestudy_16/DelaySwitch104 ==
  state Operation
  state Sending
  (default) -> Operation : {i=0;}
  (junction 7) -> Operation [order 2]
  Sending -> Operation : after(delay_array(i),msec)
      | {receive(inMsg);outMsg.data=0;send(outMsg);}
  Operation -> (junction 7) : inMsg{i = i + 1;}
  (junction 7) -> Sending [order 1] : [switch_array(i)==0]
  data: switch_array input; delay_array input; outMsg output; inMsg input; i local

== stateflow chart orion_casestudy_16/DelaySwitch105 ==
  state Operation
  state Sending
  (default) -> Operation : {i=0;}
  (junction 7) -> Operation [order 2]
  Sending -> Operation : after(delay_array(i),msec)
      | {receive(inMsg);outMsg.data=0;send(outMsg);}
  Operation -> (junction 7) : inMsg{i = i + 1;}
  (junction 7) -> Sending [order 1] : [switch_array(i)==0]
  data: switch_array input; delay_array input; outMsg output; inMsg input; i local

== stateflow chart orion_casestudy_16/DelaySwitch106 ==
  state Operation
  state Sending
  (default) -> Operation : {i=0;}
  (junction 7) -> Operation [order 2]
  Sending -> Operation : after(delay_array(i),msec)
      | {receive(inMsg);outMsg.data=0;send(outMsg);}
  Operation -> (junction 7) : inMsg{i = i + 1;}
  (junction 7) -> Sending [order 1] : [switch_array(i)==0]
  data: switch_array input; delay_array input; outMsg output; inMsg input; i local

== stateflow chart orion_casestudy_16/DelaySwitch107 ==
  state Operation
  state Sending
  (default) -> Operation : {i=0;}
  (junction 7) -> Operation [order 2]
  Sending -> Operation : after(delay_array(i),msec)
      | {receive(inMsg);outMsg.data=0;send(outMsg);}
  Operation -> (junction 7) : inMsg{i = i + 1;}
  (junction 7) -> Sending [order 1] : [switch_array(i)==0]
  data: switch_array input; delay_array input; outMsg output; inMsg input; i local

== stateflow chart orion_casestudy_16/DelaySwitch108 ==
  state Operation
  state Sending
  (default) -> Operation : {i=0;}
  (junction 7) -> Operation [order 2]
  Sending -> Operation : after(delay_array(i),msec)
      | {receive(inMsg);outMsg.data=0;send(outMsg);}
  Operation -> (junction 7) : inMsg{i = i + 1;}
  (junction 7) -> Sending [order 1] : [switch_array(i)==0]
  data: switch_array input; delay_array input; outMsg output; inMsg input; i local

== stateflow chart orion_casestudy_16/DelaySwitch109 ==
  state Operation
  state Sending
  (default) -> Operation : {i=0;}
  (junction 7) -> Operation [order 2]
  Sending -> Operation : after(delay_array(i),msec)
      | {receive(inMsg);outMsg.data=0;send(outMsg);}
  Operation -> (junction 7) : inMsg{i = i + 1;}
  (junction 7) -> Sending [order 1] : [switch_array(i)==0]
  data: switch_array input; delay_array input; outMsg output; inMsg input; i local

== stateflow chart orion_casestudy_16/DelaySwitch110 ==
  state Operation
  state Sending
  (default) -> Operation : {i=0;}
  (junction 7) -> Operation [order 2]
  Sending -> Operation : after(delay_array(i),msec)
      | {receive(inMsg);outMsg.data=0;send(outMsg);}
  Operation -> (junction 7) : inMsg{i = i + 1;}
  (junction 7) -> Sending [order 1] : [switch_array(i)==0]
  data: switch_array input; delay_array input; outMsg output; inMsg input; i local

== stateflow chart orion_casestudy_16/DelaySwitch111 ==
  state Operation
  state Sending
  (default) -> Operation : {i=0;}
  (junction 7) -> Operation [order 2]
  Sending -> Operation : after(delay_array(i),msec)
      | {receive(inMsg);outMsg.data=0;send(outMsg);}
  Operation -> (junction 7) : inMsg{i = i + 1;}
  (junction 7) -> Sending [order 1] : [switch_array(i)==0]
  data: switch_array input; delay_array input; outMsg output; inMsg input; i local

== stateflow chart orion_casestudy_16/DelaySwitch112 ==
  state Operation
  state Sending
  (default) -> Operation : {i=0;}
  (junction 7) -> Operation [order 2]
  Sending -> Operation : after(delay_array(i),msec)
      | {receive(inMsg);outMsg.data=0;send(outMsg);}
  Operation -> (junction 7) : inMsg{i = i + 1;}
  (junction 7) -> Sending [order 1] : [switch_array(i)==0]
  data: switch_array input; delay_array input; outMsg output; inMsg input; i local

== stateflow chart orion_casestudy_16/DelaySwitch113 ==
  state Operation
  state Sending
  (default) -> Operation : {i=0;}
  (junction 7) -> Operation [order 2]
  Sending -> Operation : after(delay_array(i),msec)
      | {receive(inMsg);outMsg.data=0;send(outMsg);}
  Operation -> (junction 7) : inMsg{i = i + 1;}
  (junction 7) -> Sending [order 1] : [switch_array(i)==0]
  data: switch_array input; delay_array input; outMsg output; inMsg input; i local

== stateflow chart orion_casestudy_16/DelaySwitch114 ==
  state Operation
  state Sending
  (default) -> Operation : {i=0;}
  (junction 7) -> Operation [order 2]
  Sending -> Operation : after(delay_array(i),msec)
      | {receive(inMsg);outMsg.data=0;send(outMsg);}
  Operation -> (junction 7) : inMsg{i = i + 1;}
  (junction 7) -> Sending [order 1] : [switch_array(i)==0]
  data: switch_array input; delay_array input; outMsg output; inMsg input; i local

== stateflow chart orion_casestudy_16/DelaySwitch115 ==
  state Operation
  state Sending
  (default) -> Operation : {i=0;}
  (junction 7) -> Operation [order 2]
  Sending -> Operation : after(delay_array(i),msec)
      | {receive(inMsg);outMsg.data=0;send(outMsg);}
  Operation -> (junction 7) : inMsg{i = i + 1;}
  (junction 7) -> Sending [order 1] : [switch_array(i)==0]
  data: switch_array input; delay_array input; outMsg output; inMsg input; i local

== stateflow chart orion_casestudy_16/DelaySwitch116 ==
  state Operation
  state Sending
  (default) -> Operation : {i=0;}
  (junction 7) -> Operation [order 2]
  Sending -> Operation : after(delay_array(i),msec)
      | {receive(inMsg);outMsg.data=0;send(outMsg);}
  Operation -> (junction 7) : inMsg{i = i + 1;}
  (junction 7) -> Sending [order 1] : [switch_array(i)==0]
  data: switch_array input; delay_array input; outMsg output; inMsg input; i local

== stateflow chart orion_casestudy_16/DelaySwitch117 ==
  state Operation
  state Sending
  (default) -> Operation : {i=0;}
  (junction 7) -> Operation [order 2]
  Sending -> Operation : after(delay_array(i),msec)
      | {receive(inMsg);outMsg.data=0;send(outMsg);}
  Operation -> (junction 7) : inMsg{i = i + 1;}
  (junction 7) -> Sending [order 1] : [switch_array(i)==0]
  data: switch_array input; delay_array input; outMsg output; inMsg input; i local

== stateflow chart orion_casestudy_16/DelaySwitch118 ==
  state Operation
  state Sending
  (default) -> Operation : {i=0;}
  (junction 7) -> Operation [order 2]
  Sending -> Operation : after(delay_array(i),msec)
      | {receive(inMsg);outMsg.data=0;send(outMsg);}
  Operation -> (junction 7) : inMsg{i = i + 1;}
  (junction 7) -> Sending [order 1] : [switch_array(i)==0]
  data: switch_array input; delay_array input; outMsg output; inMsg input; i local

== stateflow chart orion_casestudy_16/DelaySwitch119 ==
  state Operation
  state Sending
  (default) -> Operation : {i=0;}
  (junction 7) -> Operation [order 2]
  Sending -> Operation : after(delay_array(i),msec)
      | {receive(inMsg);outMsg.data=0;send(outMsg);}
  Operation -> (junction 7) : inMsg{i = i + 1;}
  (junction 7) -> Sending [order 1] : [switch_array(i)==0]
  data: switch_array input; delay_array input; outMsg output; inMsg input; i local

== stateflow chart orion_casestudy_16/DelaySwitch120 ==
  state Operation
  state Sending
  (default) -> Operation : {i=0;}
  (junction 7) -> Operation [order 2]
  Sending -> Operation : after(delay_array(i),msec)
      | {receive(inMsg);outMsg.data=0;send(outMsg);}
  Operation -> (junction 7) : inMsg{i = i + 1;}
  (junction 7) -> Sending [order 1] : [switch_array(i)==0]
  data: switch_array input; delay_array input; outMsg output; inMsg input; i local

== stateflow chart orion_casestudy_16/DelaySwitch121 ==
  state Operation
  state Sending
  (default) -> Operation : {i=0;}
  (junction 7) -> Operation [order 2]
  Sending -> Operation : after(delay_array(i),msec)
      | {receive(inMsg);outMsg.data=0;send(outMsg);}
  Operation -> (junction 7) : inMsg{i = i + 1;}
  (junction 7) -> Sending [order 1] : [switch_array(i)==0]
  data: switch_array input; delay_array input; outMsg output; inMsg input; i local

== stateflow chart orion_casestudy_16/DelaySwitch122 ==
  state Operation
  state Sending
  (default) -> Operation : {i=0;}
  (junction 7) -> Operation [order 2]
  Sending -> Operation : after(delay_array(i),msec)
      | {receive(inMsg);outMsg.data=0;send(outMsg);}
  Operation -> (junction 7) : inMsg{i = i + 1;}
  (junction 7) -> Sending [order 1] : [switch_array(i)==0]
  data: switch_array input; delay_array input; outMsg output; inMsg input; i local

== stateflow chart orion_casestudy_16/DelaySwitch123 ==
  state Operation
  state Sending
  (default) -> Operation : {i=0;}
  (junction 7) -> Operation [order 2]
  Sending -> Operation : after(delay_array(i),msec)
      | {receive(inMsg);outMsg.data=0;send(outMsg);}
  Operation -> (junction 7) : inMsg{i = i + 1;}
  (junction 7) -> Sending [order 1] : [switch_array(i)==0]
  data: switch_array input; delay_array input; outMsg output; inMsg input; i local

== stateflow chart orion_casestudy_16/DelaySwitch124 ==
  state Operation
  state Sending
  (default) -> Operation : {i=0;}
  (junction 7) -> Operation [order 2]
  Sending -> Operation : after(delay_array(i),msec)
      | {receive(inMsg);outMsg.data=0;send(outMsg);}
  Operation -> (junction 7) : inMsg{i = i + 1;}
  (junction 7) -> Sending [order 1] : [switch_array(i)==0]
  data: switch_array input; delay_array input; outMsg output; inMsg input; i local

== stateflow chart orion_casestudy_16/DelaySwitch125 ==
  state Operation
  state Sending
  (default) -> Operation : {i=0;}
  (junction 7) -> Operation [order 2]
  Sending -> Operation : after(delay_array(i),msec)
      | {receive(inMsg);outMsg.data=0;send(outMsg);}
  Operation -> (junction 7) : inMsg{i = i + 1;}
  (junction 7) -> Sending [order 1] : [switch_array(i)==0]
  data: switch_array input; delay_array input; outMsg output; inMsg input; i local

== stateflow chart orion_casestudy_16/DelaySwitch126 ==
  state Operation
  state Sending
  (default) -> Operation : {i=0;}
  (junction 7) -> Operation [order 2]
  Sending -> Operation : after(delay_array(i),msec)
      | {receive(inMsg);outMsg.data=0;send(outMsg);}
  Operation -> (junction 7) : inMsg{i = i + 1;}
  (junction 7) -> Sending [order 1] : [switch_array(i)==0]
  data: switch_array input; delay_array input; outMsg output; inMsg input; i local

== stateflow chart orion_casestudy_16/DelaySwitch127 ==
  state Operation
  state Sending
  (default) -> Operation : {i=0;}
  (junction 7) -> Operation [order 2]
  Sending -> Operation : after(delay_array(i),msec)
      | {receive(inMsg);outMsg.data=0;send(outMsg);}
  Operation -> (junction 7) : inMsg{i = i + 1;}
  (junction 7) -> Sending [order 1] : [switch_array(i)==0]
  data: switch_array input; delay_array input; outMsg output; inMsg input; i local

== stateflow chart orion_casestudy_16/DelaySwitch7 ==
  state Operation
  state Sending
  (default) -> Operation : {i=0;}
  (junction 7) -> Operation [order 2]
  Sending -> Operation : after(delay_array(i),msec)
      | {receive(inMsg);outMsg.data=0;send(outMsg);}
  Operation -> (junction 7) : inMsg{i = i + 1;}
  (junction 7) -> Sending [order 1] : [switch_array(i)==0]
  data: switch_array input; delay_array input; outMsg output; inMsg input; i local

== stateflow chart orion_casestudy_16/DelaySwitch128 ==
  state Operation
  state Sending
  (default) -> Operation : {i=0;}
  (junction 7) -> Operation [order 2]
  Sending -> Operation : after(delay_array(i),msec)
      | {receive(inMsg);outMsg.data=0;send(outMsg);}
  Operation -> (junction 7) : inMsg{i = i + 1;}
  (junction 7) -> Sending [order 1] : [switch_array(i)==0]
  data: switch_array input; delay_array input; outMsg output; inMsg input; i local
